simulink model "MIL_SIM"  (R2018b)
settings: Solver=FixedStepDiscrete  StartTime=0.0  StopTime=1000  FixedStep=0.002  RelTol=1e-3
undefined symbols (not defined in the file): cmd_1, cmd_2, DiscIntNeverNeededParam, ls_lr, ls_ud, mode, rs_lr, rs_ud, serial, timestamp, Ts
libraries: vrlib x2, instrumentlib x2, aerolibfltsims x2, aerolibutil x2, simulink x1, aerolibanimutils x1
settings Model: Creator=zouji  LastModifiedBy=zouji
settings OptimizationCC: DefaultParameterBehavior=Inlined  DefaultUnderspecifiedDataType=single  EnhancedBackFolding=on  PassReuseOutputArgsAs=Individual arguments  OptimizeBlockOrder=speed  DifferentSizesBufferReuse=on  OptimizationCustomize=off
settings DebuggingCC: UnderspecifiedInitializationDetection=Classic  MergeDetectMultiDrivingBlocksExec=none  ParameterTunabilityLossMsg=error
settings HardwareCC: ProdBitPerPointer=32  ProdBitPerSizeT=32  ProdBitPerPtrDiffT=32  ProdLargestAtomicInteger=Long  ProdLargestAtomicFloat=Double  ProdWordSize=32  ProdHWDeviceType=ARM Compatible->ARM Cortex
settings ModelReferenceCC: UpdateModelReferenceTargets=IfOutOfDate  PropagateSignalLabelsOutOfModel=off
settings SFSimCC: MATLABDynamicMemAlloc=off
settings RTWCC: SystemTargetFile=ert.tlc  GenCodeOnly=on  TemplateMakefile=ert_default_tmf  GenerateReport=on  IncludeHyperlinkInReport=on  LaunchReport=on  GenerateTraceInfo=on  GenerateTraceReport=on  GenerateTraceReportSl=on  GenerateTraceReportSf=on  GenerateTraceReportEml=on
settings CodeAppCC: ForceParamTrailComments=on  IgnoreCustomStorageClasses=off  OperatorAnnotations=on  SimulinkDataObjDesc=on  SFDataObjDesc=on  InsertBlockDesc=on
settings ERTTargetCC: TargetLangStandard=C99 (ISO)  GenerateSampleERTMain=on  InlinedParameterPlacement=NonHierarchical  ERTCustomFileTemplate=example_file_process.tlc

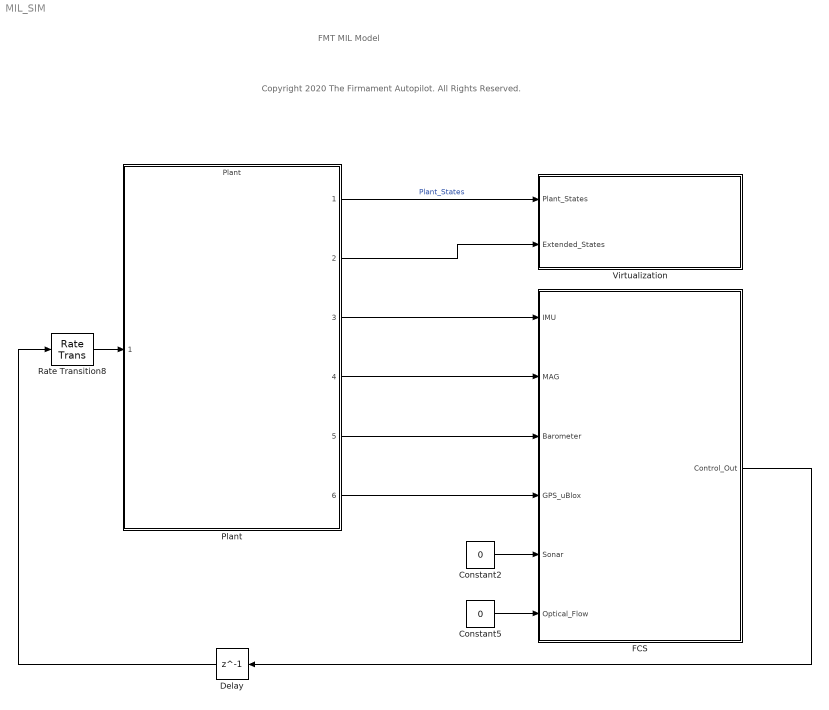
== system MIL_SIM ==
  note: FMT MIL Model
  note: Copyright 2020 The Firmament Autopilot. All Rights Reserved.
  Constant2 : Constant  Value=0  OutDataTypeStr=Bus: Sonar_Bus
  Constant5 : Constant  Value=0  OutDataTypeStr=Bus: Optical_Flow_Bus
  Delay : Delay  DelayLength=1
  FCS : Subsystem
  Plant : ModelReference  ModelNameDialog=Plant.slx  ModelReferenceVersion=1.542
  Rate Transition8 : RateTransition  OutPortSampleTime=PLANT_CONST.dt
  Virtualization : Subsystem  TreatAsAtomicUnit=on
  wires:
  Plant/1 -> Virtualization/1(Plant_States)  "Plant_States"
  Delay/1 -> Rate Transition8/1
  Rate Transition8/1 -> Plant/1
  Plant/2 -> Virtualization/2(Extended_States)
  Plant/3 -> FCS/1(IMU)
  Plant/4 -> FCS/2(MAG)
  Plant/5 -> FCS/3(Barometer)
  FCS/1(Control_Out) -> Delay/1
  Constant2/1 -> FCS/5(Sonar)
  Constant5/1 -> FCS/6(Optical_Flow)
  Plant/6 -> FCS/4(GPS_uBlox)

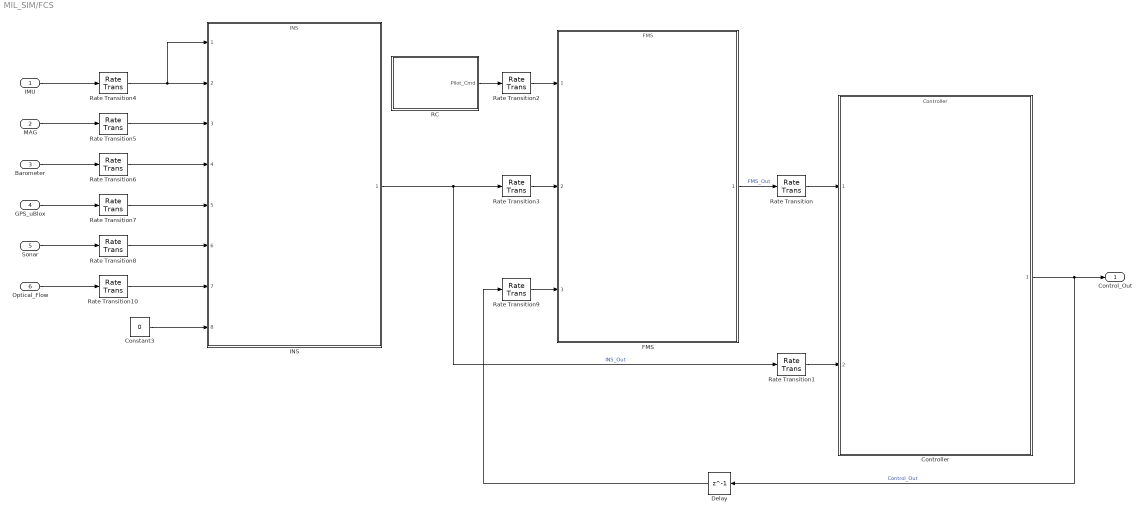
== system MIL_SIM/FCS ==
  IMU : Inport
  MAG : Inport  Port=2
  Barometer : Inport  Port=3
  GPS_uBlox : Inport  Port=4
  Sonar : Inport  Port=5
  Optical_Flow : Inport  Port=6
  Constant3 : Constant  Value=0  OutDataTypeStr=uint8
  Controller : ModelReference  ModelNameDialog=Controller.slx  ModelReferenceVersion=1.754
  Delay : Delay  DelayLength=1
  FMS : ModelReference  ModelNameDialog=FMS.slx  ModelReferenceVersion=1.935
  INS : ModelReference  ModelNameDialog=INS.slx  ModelReferenceVersion=1.2687
  RC : Subsystem  VariantControlMode=Label  Variant=on  VariantControl=Variant1  LabelModeActiveChoice=JOYSTICK_INPUT
  Rate Transition : RateTransition  OutPortSampleTime=CONTROL_CONST.dt
  Rate Transition1 : RateTransition  OutPortSampleTime=CONTROL_CONST.dt
  Rate Transition{4..8,10} (6 alike) : RateTransition  OutPortSampleTime=INS_CONST.dt
  Rate Transition2 : RateTransition  OutPortSampleTime=FMS_CONST.dt
  Rate Transition3 : RateTransition  OutPortSampleTime=FMS_CONST.dt
  Rate Transition9 : RateTransition  OutPortSampleTime=FMS_CONST.dt
  Control_Out : Outport
  wires:
  INS/1 -> Rate Transition3/1, Rate Transition1/1  "INS_Out"
  Constant3/1 -> INS/8
  Rate Transition2/1 -> FMS/1
  Rate Transition4/1 -> INS/1, INS/2
  Rate Transition/1 -> Controller/1
  Rate Transition1/1 -> Controller/2
  RC/1(" Pilot_Cmd") -> Rate Transition2/1
  Sonar/1 -> Rate Transition8/1
  GPS_uBlox/1 -> Rate Transition7/1
  FMS/1 -> Rate Transition/1  "FMS_Out"
  Rate Transition6/1 -> INS/4
  Rate Transition5/1 -> INS/3
  Barometer/1 -> Rate Transition6/1
  Rate Transition3/1 -> FMS/2
  Rate Transition10/1 -> INS/7
  MAG/1 -> Rate Transition5/1
  Rate Transition9/1 -> FMS/3
  Controller/1 -> Delay/1, Control_Out/1  "Control_Out"
  IMU/1 -> Rate Transition4/1
  Delay/1 -> Rate Transition9/1
  Rate Transition8/1 -> INS/6
  Optical_Flow/1 -> Rate Transition10/1
  Rate Transition7/1 -> INS/5

== system MIL_SIM/Virtualization ==
  Plant_States : Inport
  Extended_States : Inport  Port=2
  3D_Visualization : Subsystem  VariantControlMode=Label  Variant=on  LabelModeActiveChoice=Matlab_3D
  Simulation Pace : aerolibanimutils/Simulation Pace  SimulationPace=1  SleepMode=Auto  OutputPaceError=off  SampleTime=-1
  wires:
  Plant_States/1 -> 3D_Visualization/1(Plant_States)
  Extended_States/1 -> 3D_Visualization/2(Extended_States)

== system MIL_SIM/FCS/RC ==
  Joystick : Subsystem  VariantControl=JOYSTICK_INPUT
  Mavlink : Subsystem  VariantControl=MAVLINK_INPUT
  " Pilot_Cmd" : Outport

== system MIL_SIM/Virtualization/3D_Visualization ==
  Plant_States : Inport
  Extended_States : Inport  Port=2
  Flightgear : Subsystem  VariantControl=Flightgear
  Matlab_3D : Subsystem  VariantControl=Matlab_3D

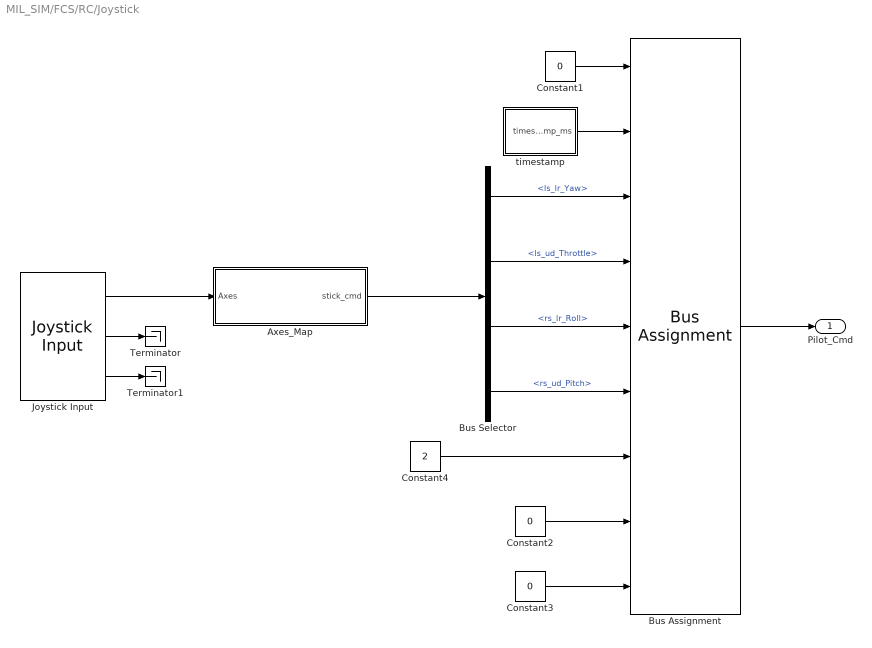
== system MIL_SIM/FCS/RC/Joystick ==
  Axes_Map : Subsystem
  Bus Assignment : BusAssignment  AssignedSignals=timestamp,ls_lr,ls_ud,rs_lr,rs_ud,mode,cmd_1,cmd_2
  Bus Selector : BusSelector  OutputSignals=ls_lr_Yaw,ls_ud_Throttle,rs_lr_Roll,rs_ud_Pitch
  Constant1 : Constant  Value=0  OutDataTypeStr=Bus: Pilot_Cmd_Bus
  Constant2 : Constant  Value=0  OutDataTypeStr=Inherit: Inherit via back propagation
  Constant3 : Constant  Value=0  OutDataTypeStr=Inherit: Inherit via back propagation
  Constant4 : Constant  Value=2  OutDataTypeStr=Inherit: Inherit via back propagation  SampleTime=-1
  Joystick Input : vrlib/Joystick Input  joyid=1  adjustports=on  forcefeed=off
      settings: SourceProductBaseCode=VR
  Terminator : Terminator
  Terminator1 : Terminator
  timestamp : Subsystem  mask{sample_time=2}
      mask prompts: sample_time "sample time (ms)"
  Pilot_Cmd : Outport  OutDataTypeStr=Bus: Pilot_Cmd_Bus
  wires:
  Constant1/1 -> Bus Assignment/1
  Constant2/1 -> Bus Assignment/8
  timestamp/1(timestamp_ms) -> Bus Assignment/2
  Bus Selector/2 -> Bus Assignment/4  "<ls_ud_Throttle>"
  Bus Selector/3 -> Bus Assignment/5  "<rs_lr_Roll>"
  Axes_Map/1(stick_cmd) -> Bus Selector/1
  Bus Selector/1 -> Bus Assignment/3  "<ls_lr_Yaw>"
  Constant3/1 -> Bus Assignment/9
  Bus Assignment/1 -> Pilot_Cmd/1
  Bus Selector/4 -> Bus Assignment/6  "<rs_ud_Pitch>"
  Constant4/1 -> Bus Assignment/7
  Joystick Input/1 -> Axes_Map/1(Axes)
  Joystick Input/2 -> Terminator/1
  Joystick Input/3 -> Terminator1/1

== system MIL_SIM/FCS/RC/Mavlink ==
  Bus Creator : BusCreator  Inputs=8
  Bus Selector : BusSelector  OutputSignals=timestamp,ls_lr,ls_ud,rs_lr,rs_ud,mode,command_1,command_2
  Display : Display
  MAVLink Decoder : S-Function  FunctionName=sfun_decode_mavlink  SFunctionDeploymentMode=off  EnableBusSupport=off
  Serial Configuration : instrumentlib/Serial Configuration  Priority=-200000  ComPortMenu=<Please select a port...>  ComPort=COM6  ObjConstructor=serial('COM6');  BaudRate=115200  DataBits=8  Parity=none  StopBits=1  FlowControl=none  Timeout=10  ByteOrder=LittleEndian
  Serial Receive : instrumentlib/Serial Receive  ComPortMenu=<Please select a port...>  ComPort=COM6  ObjConstructor=serial('COM6');  Terminator=<none>  DataSize=280  DataType=uint8  EnableBlockingMode=off  ActionDataUnavailable=Output last received value  CustomValue=0  SampleTime=-1
  Pilot_Cmd : Outport
  wires:
  Serial Receive/1 -> MAVLink Decoder/1
  Serial Receive/2 -> Display/1
  MAVLink Decoder/1 -> Bus Selector/1
  Bus Selector/1 -> Bus Creator/1  "<timestamp>"
  Bus Selector/2 -> Bus Creator/2  "<ls_lr>"
  Bus Selector/3 -> Bus Creator/3  "<ls_ud>"
  Bus Selector/4 -> Bus Creator/4  "<rs_lr>"
  Bus Selector/5 -> Bus Creator/5  "<rs_ud>"
  Bus Selector/6 -> Bus Creator/6  "<mode>"
  Bus Selector/7 -> Bus Creator/7  "<command_1>"
  Bus Selector/8 -> Bus Creator/8  "<command_2>"
  Bus Creator/1 -> Pilot_Cmd/1

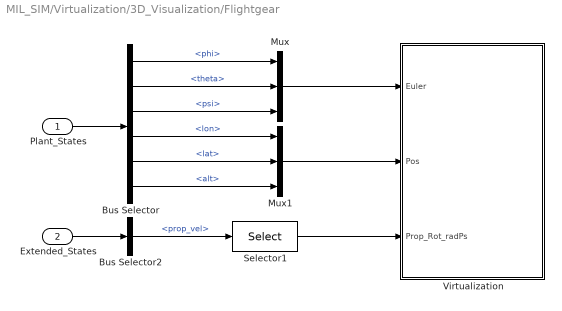
== system MIL_SIM/Virtualization/3D_Visualization/Flightgear ==
  Plant_States : Inport
  Extended_States : Inport  Port=2
  Bus Selector : BusSelector  OutputSignals=phi,theta,psi,lon,lat,alt
  Bus Selector2 : BusSelector  OutputSignals=prop_vel
  Mux : Mux  Inputs=3
  Mux1 : Mux  Inputs=3
  Selector1 : Selector  InputPortWidth=8  IndexOptions=Index vector (dialog)  Indices=[1:4]  OutputSizes=1
  Virtualization : Subsystem
  wires:
  Selector1/1 -> Virtualization/3(Prop_Rot_radPs)
  Mux/1 -> Virtualization/1(Euler)
  Mux1/1 -> Virtualization/2(Pos)
  Bus Selector2/1 -> Selector1/1  "<prop_vel>"
  Bus Selector/5 -> Mux1/2  "<lat>"
  Extended_States/1 -> Bus Selector2/1
  Plant_States/1 -> Bus Selector/1
  Bus Selector/2 -> Mux/2  "<theta>"
  Bus Selector/1 -> Mux/1  "<phi>"
  Bus Selector/6 -> Mux1/3  "<alt>"
  Bus Selector/4 -> Mux1/1  "<lon>"
  Bus Selector/3 -> Mux/3  "<psi>"

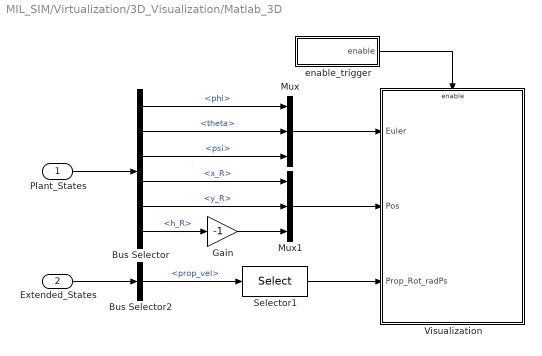
== system MIL_SIM/Virtualization/3D_Visualization/Matlab_3D ==
  Plant_States : Inport
  Extended_States : Inport  Port=2
  Bus Selector : BusSelector  OutputSignals=phi,theta,psi,x_R,y_R,h_R
  Bus Selector2 : BusSelector  OutputSignals=prop_vel
  Gain : Gain  Gain=-1
  Mux : Mux  Inputs=3
  Mux1 : Mux  Inputs=3
  Selector1 : Selector  InputPortWidth=8  IndexOptions=Index vector (dialog)  Indices=[1:4]  OutputSizes=1
  Visualization : Subsystem
  enable_trigger : Subsystem
  wires:
  Bus Selector/6 -> Gain/1  "<h_R>"
  Bus Selector/3 -> Mux/3  "<psi>"
  Bus Selector/4 -> Mux1/1  "<x_R>"
  Bus Selector2/1 -> Selector1/1  "<prop_vel>"
  Bus Selector/5 -> Mux1/2  "<y_R>"
  Bus Selector/1 -> Mux/1  "<phi>"
  Selector1/1 -> Visualization/3(Prop_Rot_radPs)
  Bus Selector/2 -> Mux/2  "<theta>"
  Mux/1 -> Visualization/1(Euler)
  Mux1/1 -> Visualization/2(Pos)
  Extended_States/1 -> Bus Selector2/1
  Plant_States/1 -> Bus Selector/1
  Gain/1 -> Mux1/3
  enable_trigger/1(enable) -> Visualization/Enable

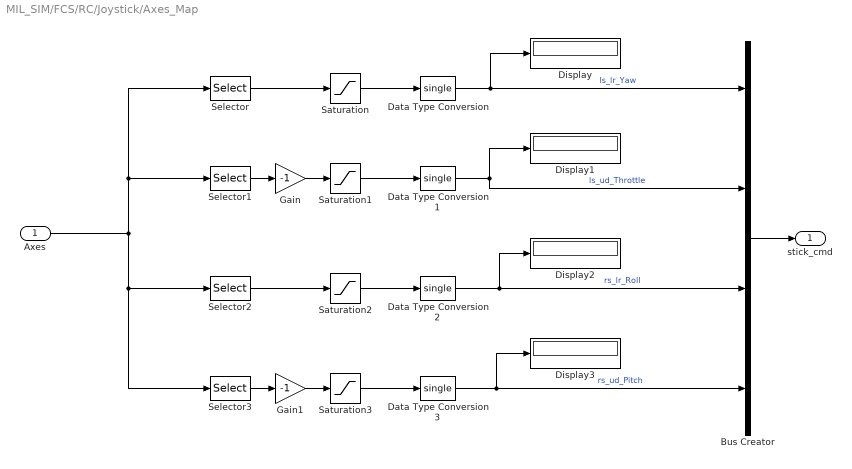
== system MIL_SIM/FCS/RC/Joystick/Axes_Map ==
  Axes : Inport
  Bus Creator : BusCreator  Inputs=4
  Data Type Conversion{,1..3} (4 alike) : DataTypeConversion  OutDataTypeStr=single
  Display{,1..3} (4 alike) : Display
  Gain : Gain  Gain=-1  OutDataTypeStr=Inherit: Same as input
  Gain1 : Gain  Gain=-1  OutDataTypeStr=Inherit: Same as input
  Saturation{,1..3} (4 alike) : Saturate  UpperLimit=1  LowerLimit=-1
  Selector : Selector  InputPortWidth=5  IndexOptions=Index vector (dialog)  Indices=1  OutputSizes=1
  Selector1 : Selector  InputPortWidth=5  IndexOptions=Index vector (dialog)  Indices=2  OutputSizes=1
  Selector2 : Selector  InputPortWidth=5  IndexOptions=Index vector (dialog)  Indices=4  OutputSizes=1
  Selector3 : Selector  InputPortWidth=5  IndexOptions=Index vector (dialog)  Indices=5  OutputSizes=1
  stick_cmd : Outport
  wires:
  Data Type Conversion1/1 -> Display1/1, Bus Creator/2  "ls_ud_Throttle"
  Data Type Conversion2/1 -> Display2/1, Bus Creator/3  "rs_lr_Roll"
  Gain/1 -> Saturation1/1
  Gain1/1 -> Saturation3/1
  Axes/1 -> Selector3/1, Selector2/1, Selector/1, Selector1/1
  Data Type Conversion3/1 -> Display3/1, Bus Creator/4  "rs_ud_Pitch"
  Data Type Conversion/1 -> Display/1, Bus Creator/1  "ls_lr_Yaw"
  Bus Creator/1 -> stick_cmd/1
  Saturation/1 -> Data Type Conversion/1
  Saturation1/1 -> Data Type Conversion1/1
  Saturation2/1 -> Data Type Conversion2/1
  Saturation3/1 -> Data Type Conversion3/1
  Selector/1 -> Saturation/1
  Selector1/1 -> Gain/1
  Selector2/1 -> Saturation2/1
  Selector3/1 -> Gain1/1

== system MIL_SIM/FCS/RC/Joystick/timestamp ==
  Constant : Constant  Value=sample_time
  Data Type Conversion : DataTypeConversion  OutDataTypeStr=uint32
  Discrete-Time Integrator : DiscreteIntegrator  IntegratorMethod=Accumulation: Forward Euler  SampleTime=-1  ICPrevOutput=DiscIntNeverNeededParam  ICPrevScaledInput=DiscIntNeverNeededParam
  timestamp_ms : Outport
  wires:
  Discrete-Time Integrator/1 -> Data Type Conversion/1
  Constant/1 -> Discrete-Time Integrator/1
  Data Type Conversion/1 -> timestamp_ms/1

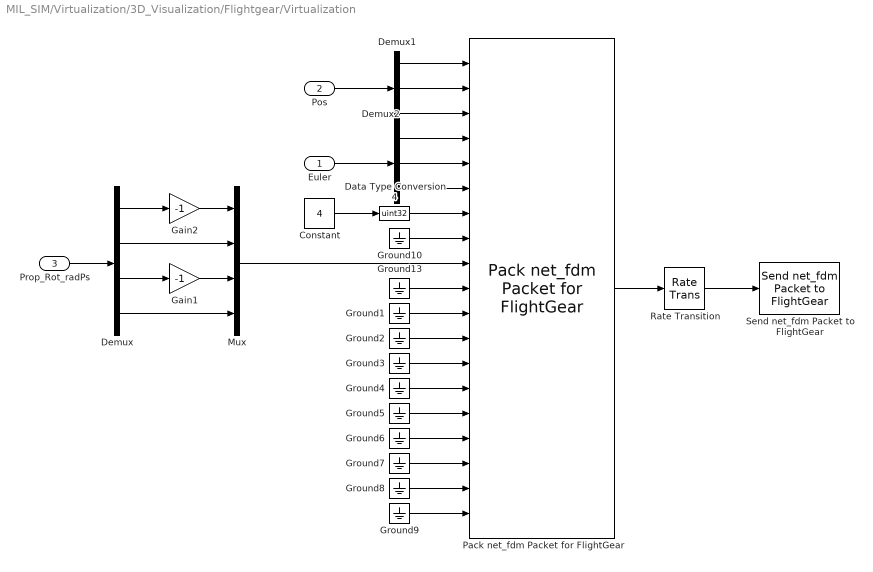
== system MIL_SIM/Virtualization/3D_Visualization/Flightgear/Virtualization ==
  Euler : Inport
  Pos : Inport  Port=2
  Prop_Rot_radPs : Inport  Port=3
  Constant : Constant  Value=4
  Data Type Conversion4 : DataTypeConversion  OutDataTypeStr=uint32
  Demux : Demux
  Demux1 : Demux  Outputs=3
  Demux2 : Demux  Outputs=3
  Gain1 : Gain  Gain=-1  OutDataTypeStr=Inherit: Same as input
  Gain2 : Gain  Gain=-1  OutDataTypeStr=Inherit: Same as input
  Ground{1..10,13} (11 alike) : Ground
  Mux : Mux
  Pack net_fdm Packet for FlightGear : aerolibfltsims/Pack net_fdm Packet for FlightGear  FlightGearVersion=v2016.1  ShowPositionAttitudeInputs=on  ShowVelocityAccelerationInputs=off  ShowControlSurfacePositionInputs=off  ShowEngineFuelInputs=on  ShowLandingGearInputs=off  ShowEnvironmentInputs=off  SampleTime=1/50  packetVersion=24
      settings: SourceProductName=Aerospace Blockset  SourceProductBaseCode=AE
  Rate Transition : RateTransition
  Send net_fdm Packet to FlightGear : aerolibfltsims/Send net_fdm Packet to FlightGear  DestinationIpAddress=127.0.0.1  DestinationPort=5502  LocalIpPort=-1  varLen=off  SampleTime=1/25
      settings: SourceProductName=Aerospace Blockset  SourceProductBaseCode=AE
  wires:
  Euler/1 -> Demux2/1
  Demux/4 -> Mux/4
  Pos/1 -> Demux1/1
  Prop_Rot_radPs/1 -> Demux/1
  Demux1/1 -> Pack net_fdm Packet for FlightGear/1
  Rate Transition/1 -> Send net_fdm Packet to FlightGear/1
  Demux2/1 -> Pack net_fdm Packet for FlightGear/4
  Demux2/3 -> Pack net_fdm Packet for FlightGear/6
  Demux2/2 -> Pack net_fdm Packet for FlightGear/5
  Demux1/3 -> Pack net_fdm Packet for FlightGear/3
  Demux1/2 -> Pack net_fdm Packet for FlightGear/2
  Ground13/1 -> Pack net_fdm Packet for FlightGear/10
  Ground1/1 -> Pack net_fdm Packet for FlightGear/11
  Ground2/1 -> Pack net_fdm Packet for FlightGear/12
  Ground3/1 -> Pack net_fdm Packet for FlightGear/13
  Ground4/1 -> Pack net_fdm Packet for FlightGear/14
  Ground5/1 -> Pack net_fdm Packet for FlightGear/15
  Ground6/1 -> Pack net_fdm Packet for FlightGear/16
  Ground7/1 -> Pack net_fdm Packet for FlightGear/17
  Ground8/1 -> Pack net_fdm Packet for FlightGear/18
  Ground9/1 -> Pack net_fdm Packet for FlightGear/19
  Constant/1 -> Data Type Conversion4/1
  Data Type Conversion4/1 -> Pack net_fdm Packet for FlightGear/7
  Ground10/1 -> Pack net_fdm Packet for FlightGear/8
  Pack net_fdm Packet for FlightGear/1 -> Rate Transition/1
  Gain2/1 -> Mux/1
  Demux/1 -> Gain2/1
  Demux/2 -> Mux/2
  Demux/3 -> Gain1/1
  Mux/1 -> Pack net_fdm Packet for FlightGear/9
  Gain1/1 -> Mux/3

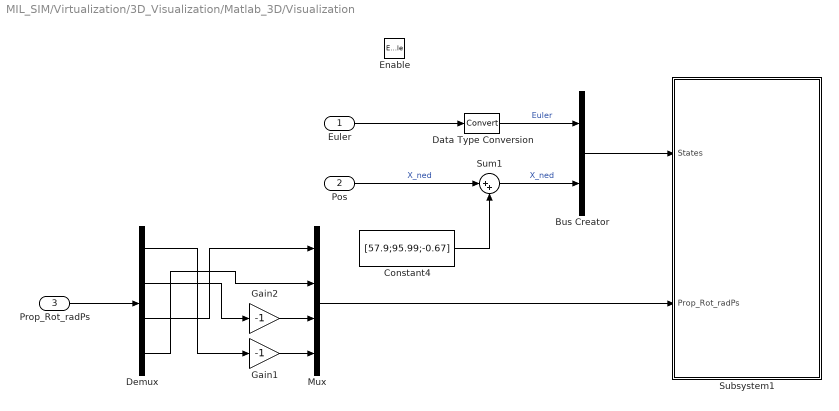
== system MIL_SIM/Virtualization/3D_Visualization/Matlab_3D/Visualization ==
  Euler : Inport
  Pos : Inport  Port=2
  Prop_Rot_radPs : Inport  Port=3
  Enable : EnablePort
  Bus Creator : BusCreator  Inputs=2
  Constant4 : Constant  Value=[57.9;95.99;-0.67]  OutDataTypeStr=Inherit: Inherit via back propagation
  Data Type Conversion : DataTypeConversion
  Demux : Demux
  Gain1 : Gain  Gain=-1  OutDataTypeStr=Inherit: Same as input
  Gain2 : Gain  Gain=-1  OutDataTypeStr=Inherit: Same as input
  Mux : Mux
  Subsystem1 : Subsystem
  Sum1 : Sum  Inputs=|++
  wires:
  Bus Creator/1 -> Subsystem1/1(States)
  Euler/1 -> Data Type Conversion/1
  Sum1/1 -> Bus Creator/2  "X_ned"
  Demux/1 -> Gain1/1
  Gain1/1 -> Mux/4
  Demux/2 -> Gain2/1
  Demux/3 -> Mux/1
  Demux/4 -> Mux/2
  Gain2/1 -> Mux/3
  Mux/1 -> Subsystem1/2(Prop_Rot_radPs)
  Constant4/1 -> Sum1/2
  Pos/1 -> Sum1/1  "X_ned"
  Data Type Conversion/1 -> Bus Creator/1  "Euler"
  Prop_Rot_radPs/1 -> Demux/1

== system MIL_SIM/Virtualization/3D_Visualization/Matlab_3D/enable_trigger ==
  Compare To Zero : simulink/Logic and Bit Operations/Compare To Zero  relop===  OutDataTypeStr=boolean
  Constant : Constant  Value=40  OutDataTypeStr=Inherit: Inherit via back propagation
  Counter : Subsystem
  Mod : Math  Operator=rem  SaturateOnIntegerOverflow=on
  enable : Outport
  wires:
  Constant/1 -> Mod/2
  Counter/1(Timestamp_ms) -> Mod/1  "timestamp"
  Mod/1 -> Compare To Zero/1
  Compare To Zero/1 -> enable/1

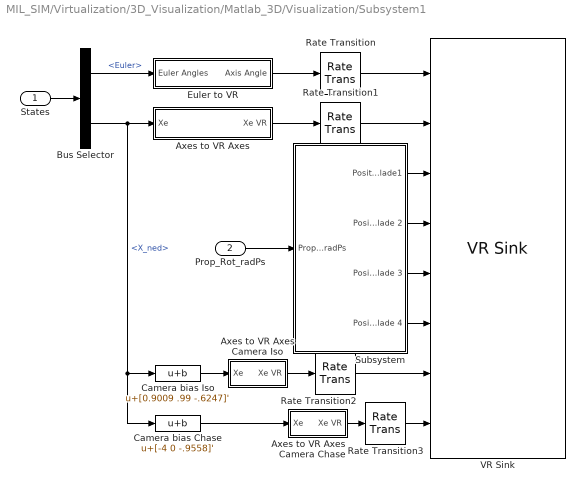
== system MIL_SIM/Virtualization/3D_Visualization/Matlab_3D/Visualization/Subsystem1 ==
  States : Inport
  Prop_Rot_radPs : Inport  Port=2
  Axes to VR Axes : Subsystem
  Axes to VR Axes Camera Chase : Subsystem
  Axes to VR Axes Camera Iso : Subsystem
  Bus Selector : BusSelector  OutputSignals=Euler,X_ned
  Camera bias Chase : Bias  Bias=[-4 0 -.9558]'
  Camera bias Iso : Bias  Bias=[0.9009 .99 -.6247]'
  Euler to VR : Subsystem
  Rate Transition{,1..3} (4 alike) : RateTransition
  Subsystem : Subsystem
  VR Sink : vrlib/VR Sink  InstantiateOnLoad=on  SampleTime=12*Ts  ViewEnable=on  RemoteChange=off  RemoteView=off  FieldsWritten=QuadBody.rotation.4.1.1.double#QuadBody.translation.3.1.1.double#Blade1.rotation.4.1.1.double#Blade3.rotation.4.1.1.double#Blade2.rotation.4.1.1.double#Blade4.rotation.4.1.1.double#IsoNoRotation.position.3.1.1.double#OnQuadNoRotation.position.3.1.1.double  WorldFileName=asbQuadcopterWorld.wrl  AutoView=on  VideoDimensions=[]  AllowVariableSize=off  FigureProperties="{'Position', 'Name', 'Viewpoint', 'CameraBound', 'CameraDirection', 'CameraPosition', 'CameraUpVector', 'ZoomFactor', 'Antialiasing', 'Headlight', 'Lighting', 'NavPanel', 'Sound', 'StatusBar', 'Stereo3D', 'Stereo3DCameraOffset', 'Stereo3DHIT', 'ToolBar', 'Textures', 'Transparency', 'Triad', 'Wireframe', 'NavZones', 'NavMode', 'NavSpeed', 'CaptureFileFormat', 'CaptureFileName', 'Record2DCompressMethod', 'Record2DCompressQuality', 'Record2D', 'Record2DFileName', 'Record2DFPS'; [5.0000000000000000e+00   9.2000000000000000e+01   5.7600000000000000e+02   3.5000000000000000e+02], '', 'Isometric - No Rotation', 'on', [0.0000000000000000e+00   0.0000000000000000e+00  -1.0000000000000000e+00], [0.0000000000000000e+00   0.0000000000000000e+00   0.0000000000000000e+00], [0.0000000000000000e+00   1.0000000000000000e+00   0.0000000000000000e+00], [1.0000000000000000e+00], 'on', 'on', 'on', 'halfbar', 'on', 'on', 'off', [1.0000000149011612e-01], [0.0000000000000000e+00], 'on', 'on', 'on', 'none', 'off', 'off', 'fly', 'normal', 'tif', '%f_anim_%n.tif', 'auto', [7.5000000000000000e+01], 'off', '%f_anim_%n.avi', 'auto'}"
      settings: SourceProductBaseCode=VR
  wires:
  Rate Transition/1 -> VR Sink/1
  Subsystem/3(Position Blade 3) -> VR Sink/5
  States/1 -> Bus Selector/1
  Subsystem/4(Position Blade 4) -> VR Sink/6
  Bus Selector/1 -> Euler to VR/1(Euler Angles)  "<Euler>"
  Camera bias Iso/1 -> Axes to VR Axes Camera Iso/1(Xe)
  Axes to VR Axes/1(Xe VR) -> Rate Transition1/1
  Rate Transition1/1 -> VR Sink/2
  Axes to VR Axes Camera Iso/1(Xe VR) -> Rate Transition2/1
  Bus Selector/2 -> Camera bias Chase/1, Camera bias Iso/1, Axes to VR Axes/1(Xe)  "<X_ned>"
  Axes to VR Axes Camera Chase/1(Xe VR) -> Rate Transition3/1
  Subsystem/2(Position Blade 2) -> VR Sink/4
  Prop_Rot_radPs/1 -> Subsystem/1(Prop_Rot_radPs)
  Subsystem/1(Position Blade1) -> VR Sink/3
  Euler to VR/1(Axis Angle) -> Rate Transition/1
  Rate Transition3/1 -> VR Sink/8
  Rate Transition2/1 -> VR Sink/7
  Camera bias Chase/1 -> Axes to VR Axes Camera Chase/1(Xe)

== system MIL_SIM/Virtualization/3D_Visualization/Matlab_3D/enable_trigger/Counter ==
  Add : Sum
  Constant : Constant  Value=2  OutDataTypeStr=uint32
  Data Type Conversion : DataTypeConversion  OutDataTypeStr=uint32
  Output : UnitDelay  InitialCondition=0.0  SampleTime=-1
  Timestamp_ms : Outport
  wires:
  Add/1 -> Output/1
  Output/1 -> Add/2, Data Type Conversion/1
  Data Type Conversion/1 -> Timestamp_ms/1  "Timestamp_ms"
  Constant/1 -> Add/1

== system MIL_SIM/Virtualization/3D_Visualization/Matlab_3D/Visualization/Subsystem1/Axes to VR Axes ==
  Xe : Inport
  Demux : Demux  Outputs=3
  Mux : Mux  Inputs=3
  rad-->deg1 : Gain  Gain=-1  SaturateOnIntegerOverflow=on  OutDataTypeStr=Inherit: Same as input  ParamDataTypeStr=Inherit: Same as input
  Xe VR : Outport
  wires:
  Xe/1 -> Demux/1
  Demux/1 -> Mux/1
  Demux/3 -> rad-->deg1/1
  Mux/1 -> Xe VR/1
  rad-->deg1/1 -> Mux/2
  Demux/2 -> Mux/3

== system MIL_SIM/Virtualization/3D_Visualization/Matlab_3D/Visualization/Subsystem1/Axes to VR Axes Camera Chase ==
  Xe : Inport
  Demux : Demux  Outputs=3
  Mux : Mux  Inputs=3
  rad-->deg1 : Gain  Gain=-1  SaturateOnIntegerOverflow=on  OutDataTypeStr=Inherit: Same as input  ParamDataTypeStr=Inherit: Same as input
  Xe VR : Outport
  wires:
  Xe/1 -> Demux/1
  Demux/1 -> Mux/1
  Demux/3 -> rad-->deg1/1
  Mux/1 -> Xe VR/1
  rad-->deg1/1 -> Mux/2
  Demux/2 -> Mux/3

== system MIL_SIM/Virtualization/3D_Visualization/Matlab_3D/Visualization/Subsystem1/Axes to VR Axes Camera Iso ==
  Xe : Inport
  Demux : Demux  Outputs=3
  Mux : Mux  Inputs=3
  rad-->deg1 : Gain  Gain=-1  SaturateOnIntegerOverflow=on  OutDataTypeStr=Inherit: Same as input  ParamDataTypeStr=Inherit: Same as input
  Xe VR : Outport
  wires:
  Demux/2 -> Mux/3
  rad-->deg1/1 -> Mux/2
  Mux/1 -> Xe VR/1
  Demux/3 -> rad-->deg1/1
  Demux/1 -> Mux/1
  Xe/1 -> Demux/1

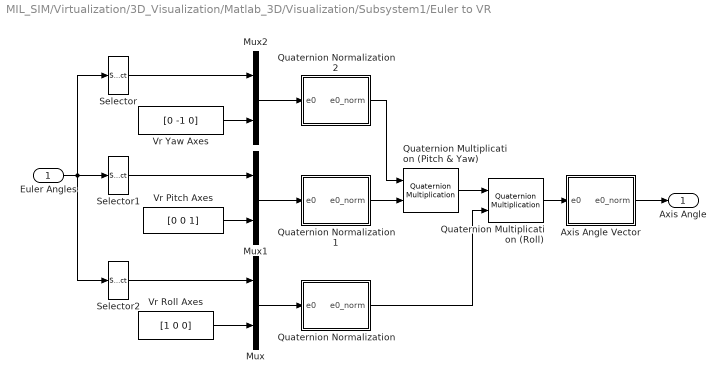
== system MIL_SIM/Virtualization/3D_Visualization/Matlab_3D/Visualization/Subsystem1/Euler to VR ==
  Euler Angles : Inport
  Axis Angle Vector : Subsystem
  Mux : Mux  Inputs=2
  Mux1 : Mux  Inputs=2
  Mux2 : Mux  Inputs=2
  Quaternion Multiplication (Pitch & Yaw) : aerolibutil/Quaternion Multiplication
  Quaternion Multiplication (Roll) : aerolibutil/Quaternion Multiplication
  Quaternion Normalization : Subsystem
  Quaternion Normalization1 : Subsystem
  Quaternion Normalization2 : Subsystem
  Selector : Selector  InputPortWidth=3  IndexOptions=Index vector (dialog)  Indices=[3]  OutputSizes=1
  Selector1 : Selector  InputPortWidth=3  IndexOptions=Index vector (dialog)  Indices=[2]  OutputSizes=1
  Selector2 : Selector  InputPortWidth=3  IndexOptions=Index vector (dialog)  Indices=[1]  OutputSizes=1
  Vr Pitch Axes : Constant  Value=[0 0 1]
  Vr Roll Axes : Constant  Value=[1 0 0]
  Vr Yaw Axes : Constant  Value=[0 -1 0]
  Axis Angle : Outport
  wires:
  Quaternion Multiplication (Roll)/1 -> Axis Angle Vector/1(e0)
  Axis Angle Vector/1(e0_norm) -> Axis Angle/1
  Quaternion Normalization/1(e0_norm) -> Quaternion Multiplication (Roll)/2
  Quaternion Normalization2/1(e0_norm) -> Quaternion Multiplication (Pitch & Yaw)/1
  Quaternion Normalization1/1(e0_norm) -> Quaternion Multiplication (Pitch & Yaw)/2
  Mux2/1 -> Quaternion Normalization2/1(e0)
  Mux1/1 -> Quaternion Normalization1/1(e0)
  Mux/1 -> Quaternion Normalization/1(e0)
  Selector/1 -> Mux2/1
  Vr Yaw Axes/1 -> Mux2/2
  Selector1/1 -> Mux1/1
  Vr Pitch Axes/1 -> Mux1/2
  Selector2/1 -> Mux/1
  Vr Roll Axes/1 -> Mux/2
  Euler Angles/1 -> Selector2/1, Selector1/1, Selector/1
  Quaternion Multiplication (Pitch & Yaw)/1 -> Quaternion Multiplication (Roll)/1

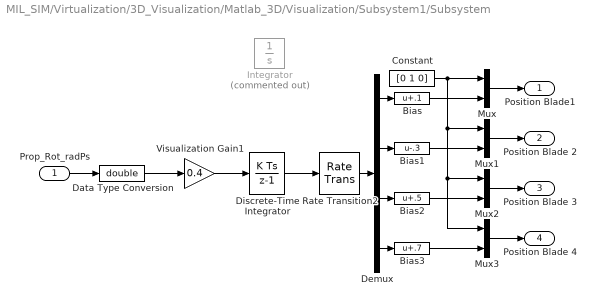
== system MIL_SIM/Virtualization/3D_Visualization/Matlab_3D/Visualization/Subsystem1/Subsystem ==
  Prop_Rot_radPs : Inport
  Bias : Bias  Bias=.1
  Bias1 : Bias  Bias=-.3
  Bias2 : Bias  Bias=.5
  Bias3 : Bias  Bias=.7
  Constant : Constant  Value=[0 1 0]
  Data Type Conversion : DataTypeConversion  OutDataTypeStr=double
  Demux : Demux
  Discrete-Time Integrator : DiscreteIntegrator  InitialCondition="[.1  .2 -.3 -.4]"  SampleTime=-1  UpperSaturationLimit=2*pi  LowerSaturationLimit=-2*pi  ICPrevOutput=DiscIntNeverNeededParam  ICPrevScaledInput=DiscIntNeverNeededParam
  Integrator : Integrator  Commented=on  InitialCondition="[.1  .2 -.3 -.4]"  WrapState=on  WrappedStateUpperValue=2*pi  WrappedStateLowerValue=-2*pi
  Mux{,1..3} (4 alike) : Mux  Inputs=2
  Rate Transition2 : RateTransition
  Visualization Gain1 : Gain  Gain=0.4
  Position Blade1 : Outport
  Position Blade 2 : Outport  Port=2
  Position Blade 3 : Outport  Port=3
  Position Blade 4 : Outport  Port=4
  wires:
  Bias3/1 -> Mux3/2
  Mux3/1 -> Position Blade 4/1
  Bias1/1 -> Mux1/2
  Bias2/1 -> Mux2/2
  Demux/2 -> Bias1/1
  Constant/1 -> Mux3/1, Mux2/1, Mux1/1, Mux/1
  Mux1/1 -> Position Blade 2/1
  Mux2/1 -> Position Blade 3/1
  Data Type Conversion/1 -> Visualization Gain1/1
  Discrete-Time Integrator/1 -> Rate Transition2/1
  Mux/1 -> Position Blade1/1
  Demux/3 -> Bias2/1
  Bias/1 -> Mux/2
  Prop_Rot_radPs/1 -> Data Type Conversion/1
  Demux/4 -> Bias3/1
  Rate Transition2/1 -> Demux/1
  Demux/1 -> Bias/1
  Visualization Gain1/1 -> Discrete-Time Integrator/1

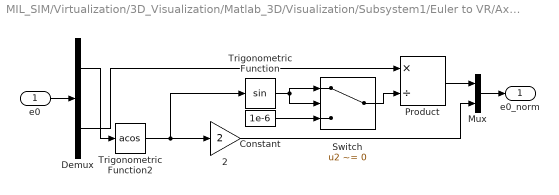
== system MIL_SIM/Virtualization/3D_Visualization/Matlab_3D/Visualization/Subsystem1/Euler to VR/Axis Angle Vector ==
  e0 : Inport
  2 : Gain  Gain=2  SaturateOnIntegerOverflow=on  OutDataTypeStr=Inherit: Same as input  ParamDataTypeStr=Inherit: Same as input
  Constant : Constant  Value=1e-6
  Demux : Demux  Outputs=[1 3 ]
  Mux : Mux  Inputs=2
  Product : Product  Inputs=*/  SaturateOnIntegerOverflow=on  InputSameDT=on  OutDataTypeStr=Inherit: Same as first input
  Switch : Switch  Criteria=u2 ~= 0
  Trigonometric Function : Trigonometry
  Trigonometric Function2 : Trigonometry  Operator=acos
  e0_norm : Outport
  wires:
  Demux/1 -> Trigonometric Function2/1
  Demux/2 -> Product/1
  Mux/1 -> e0_norm/1
  Product/1 -> Mux/1
  2/1 -> Mux/2
  Trigonometric Function/1 -> Switch/1, Switch/2
  Trigonometric Function2/1 -> Trigonometric Function/1, 2/1
  e0/1 -> Demux/1
  Constant/1 -> Switch/3
  Switch/1 -> Product/2

== system MIL_SIM/Virtualization/3D_Visualization/Matlab_3D/Visualization/Subsystem1/Euler to VR/Quaternion Normalization ==
  e0 : Inport
  1/2 : Gain  Gain=1/2  SaturateOnIntegerOverflow=on  OutDataTypeStr=Inherit: Same as input  ParamDataTypeStr=Inherit: Same as input
  Demux : Demux  Outputs=[1 3]
  Mux : Mux  Inputs=2
  Product : Product  SaturateOnIntegerOverflow=on  InputSameDT=on  OutDataTypeStr=Inherit: Same as first input
  Trigonometric Function : Trigonometry
  Trigonometric Function1 : Trigonometry  Operator=cos
  e0_norm : Outport
  wires:
  Trigonometric Function1/1 -> Mux/1
  Demux/2 -> Product/2
  Demux/1 -> 1/2/1
  Mux/1 -> e0_norm/1
  Product/1 -> Mux/2
  Trigonometric Function/1 -> Product/1
  1/2/1 -> Trigonometric Function1/1, Trigonometric Function/1
  e0/1 -> Demux/1

== system MIL_SIM/Virtualization/3D_Visualization/Matlab_3D/Visualization/Subsystem1/Euler to VR/Quaternion Normalization1 ==
  e0 : Inport
  1/2 : Gain  Gain=1/2  SaturateOnIntegerOverflow=on  OutDataTypeStr=Inherit: Same as input  ParamDataTypeStr=Inherit: Same as input
  Demux : Demux  Outputs=[1 3]
  Mux : Mux  Inputs=2
  Product : Product  SaturateOnIntegerOverflow=on  InputSameDT=on  OutDataTypeStr=Inherit: Same as first input
  Trigonometric Function : Trigonometry
  Trigonometric Function1 : Trigonometry  Operator=cos
  e0_norm : Outport
  wires:
  e0/1 -> Demux/1
  1/2/1 -> Trigonometric Function/1, Trigonometric Function1/1
  Trigonometric Function/1 -> Product/1
  Product/1 -> Mux/2
  Mux/1 -> e0_norm/1
  Demux/1 -> 1/2/1
  Demux/2 -> Product/2
  Trigonometric Function1/1 -> Mux/1

== system MIL_SIM/Virtualization/3D_Visualization/Matlab_3D/Visualization/Subsystem1/Euler to VR/Quaternion Normalization2 ==
  e0 : Inport
  1/2 : Gain  Gain=1/2  SaturateOnIntegerOverflow=on  OutDataTypeStr=Inherit: Same as input  ParamDataTypeStr=Inherit: Same as input
  Demux : Demux  Outputs=[1 3]
  Mux : Mux  Inputs=2
  Product : Product  SaturateOnIntegerOverflow=on  InputSameDT=on  OutDataTypeStr=Inherit: Same as first input
  Trigonometric Function : Trigonometry
  Trigonometric Function1 : Trigonometry  Operator=cos
  e0_norm : Outport
  wires:
  Trigonometric Function1/1 -> Mux/1
  Demux/2 -> Product/2
  Demux/1 -> 1/2/1
  Mux/1 -> e0_norm/1
  Product/1 -> Mux/2
  Trigonometric Function/1 -> Product/1
  1/2/1 -> Trigonometric Function1/1, Trigonometric Function/1
  e0/1 -> Demux/1
